simulink model "eqgraph"  (R2025b)
settings: Solver=FixedStepDiscrete  StartTime=0.0  StopTime=inf  RelTol=1e-3
undefined symbols (not defined in the file): Gain1_rt, Gain2_rt, Gain3_rt, Gain4_rt, Gain5_rt, Gain6_rt, Gain7_rt, Gain_rt
settings Model: Creator=linogarciamorales  LastModifiedBy=linogarciamorales
settings OptimizationCC: EnhancedBackFolding=on  PassReuseOutputArgsAs=Individual arguments  ZeroExternalMemoryAtStartup=off  ZeroInternalMemoryAtStartup=off  OptimizeBlockOrder=speed  DifferentSizesBufferReuse=on  OptimizationCustomize=off  EfficientTunableParamExpr=on
settings DebuggingCC: ParameterTunabilityLossMsg=error
settings HardwareCC: ProdBitPerPointer=32.0  ProdBitPerSizeT=32.0  ProdBitPerPtrDiffT=32.0  ProdLargestAtomicFloat=None  ProdIntDivRoundTo=Undefined  ProdEndianess=Unspecified  ProdWordSize=32.0  ProdHWDeviceType=Generic->32-bit Embedded Processor
settings SFSimCC: MATLABDynamicMemAlloc=off
settings RTWCC: SystemTargetFile=ert.tlc  GenCodeOnly=on  TemplateMakefile=ert_default_tmf  Description=Embedded Coder
settings CodeAppCC: ForceParamTrailComments=on  IgnoreCustomStorageClasses=off  OperatorAnnotations=on  SimulinkDataObjDesc=on  SFDataObjDesc=on  InsertBlockDesc=on
settings ERTTargetCC: InlinedParameterPlacement=Hierarchical  ERTCustomFileTemplate=example_file_process.tlc  TargetLangStandard=C99 (ISO)  SupportNonInlinedSFcns=on

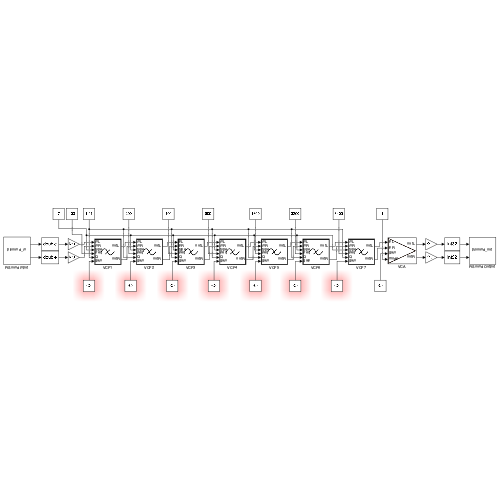
[thumbnail: Simulink's stored preview of the top-level diagram]
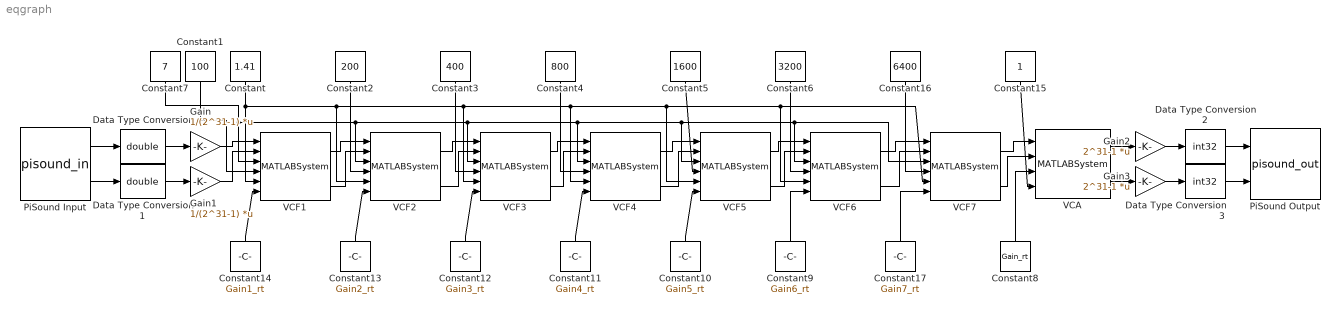
== system eqgraph ==
  Constant : Constant  Value=1.41  OutDataTypeStr=double
  Constant1 : Constant  Value=100  OutDataTypeStr=double
  Constant10 : Constant  Value=Gain5_rt  OutDataTypeStr=double
  Constant11 : Constant  Value=Gain4_rt  OutDataTypeStr=double
  Constant12 : Constant  Value=Gain3_rt  OutDataTypeStr=double
  Constant13 : Constant  Value=Gain2_rt  OutDataTypeStr=double
  Constant14 : Constant  Value=Gain1_rt  OutDataTypeStr=double
  Constant15 : Constant  OutDataTypeStr=uint8
  Constant16 : Constant  Value=6400  OutDataTypeStr=double
  Constant17 : Constant  Value=Gain7_rt  OutDataTypeStr=double
  Constant2 : Constant  Value=200  OutDataTypeStr=double
  Constant3 : Constant  Value=400  OutDataTypeStr=double
  Constant4 : Constant  Value=800  OutDataTypeStr=double
  Constant5 : Constant  Value=1600  OutDataTypeStr=double
  Constant6 : Constant  Value=3200  OutDataTypeStr=double
  Constant7 : Constant  Value=7  OutDataTypeStr=uint8
  Constant8 : Constant  Value=Gain_rt  OutDataTypeStr=double
  Constant9 : Constant  Value=Gain6_rt  OutDataTypeStr=double
  Data Type Conversion : DataTypeConversion  OutDataTypeStr=double  SaturateOnIntegerOverflow=off  RndMeth=Floor
  Data Type Conversion1 : DataTypeConversion  OutDataTypeStr=double  SaturateOnIntegerOverflow=off  RndMeth=Floor
  Data Type Conversion2 : DataTypeConversion  OutDataTypeStr=int32  SaturateOnIntegerOverflow=off  RndMeth=Floor
  Data Type Conversion3 : DataTypeConversion  OutDataTypeStr=int32  SaturateOnIntegerOverflow=off  RndMeth=Floor
  Gain : Gain  Gain=1/(2^31-1)  Multiplication=Matrix(K*u)
  Gain1 : Gain  Gain=1/(2^31-1)  Multiplication=Matrix(K*u)
  Gain2 : Gain  Gain=2^31-1  Multiplication=Matrix(K*u)
  Gain3 : Gain  Gain=2^31-1  Multiplication=Matrix(K*u)
  PiSound Input : S-Function  FunctionName=pisound_in  Parameters=48000, 128, 0  SFunctionDeploymentMode=off  EnableBusSupport=off
  PiSound Output : S-Function  FunctionName=pisound_out  Parameters=48000, 128, 0  SFunctionDeploymentMode=off  EnableBusSupport=off
  VCA : MATLABSystem  System=vca_sys  N=128  Fs=48000  bypass=uint8(0)  SimulateUsing=Code generation
      mask Type: vca_sys
  VCF1 : MATLABSystem  InitFcn=|  System=vcf_sys  N=128  Fs=48000  bypass=uint8(0)  SimulateUsing=Code generation
      | Type_rt = uint8(1);   % 1..7
      | Freq_rt = 1000;       % Hz
      | Q_rt    = 0.707;
      | Gain_rt = 0;          % dB
      mask Type: vcf_sys
  VCF2 : MATLABSystem  InitFcn=|  System=vcf_sys  N=128  Fs=48000  bypass=uint8(0)  SimulateUsing=Code generation
      | Type_rt = uint8(1);   % 1..7
      | Freq_rt = 1000;       % Hz
      | Q_rt    = 0.707;
      | Gain_rt = 0;          % dB
      mask Type: vcf_sys
  VCF3 : MATLABSystem  InitFcn=|  System=vcf_sys  N=128  Fs=48000  bypass=uint8(0)  SimulateUsing=Code generation
      | Type_rt = uint8(1);   % 1..7
      | Freq_rt = 1000;       % Hz
      | Q_rt    = 0.707;
      | Gain_rt = 0;          % dB
      mask Type: vcf_sys
  VCF4 : MATLABSystem  InitFcn=|  System=vcf_sys  N=128  Fs=48000  bypass=uint8(0)  SimulateUsing=Code generation
      | Type_rt = uint8(1);   % 1..7
      | Freq_rt = 1000;       % Hz
      | Q_rt    = 0.707;
      | Gain_rt = 0;          % dB
      mask Type: vcf_sys
  VCF5 : MATLABSystem  InitFcn=|  System=vcf_sys  N=128  Fs=48000  bypass=uint8(0)  SimulateUsing=Code generation
      | Type_rt = uint8(1);   % 1..7
      | Freq_rt = 1000;       % Hz
      | Q_rt    = 0.707;
      | Gain_rt = 0;          % dB
      mask Type: vcf_sys
  VCF6 : MATLABSystem  InitFcn=|  System=vcf_sys  N=128  Fs=48000  bypass=uint8(0)  SimulateUsing=Code generation
      | Type_rt = uint8(1);   % 1..7
      | Freq_rt = 1000;       % Hz
      | Q_rt    = 0.707;
      | Gain_rt = 0;          % dB
      mask Type: vcf_sys
  VCF7 : MATLABSystem  InitFcn=|  System=vcf_sys  N=128  Fs=48000  bypass=uint8(0)  SimulateUsing=Code generation
      | Type_rt = uint8(1);   % 1..7
      | Freq_rt = 1000;       % Hz
      | Q_rt    = 0.707;
      | Gain_rt = 0;          % dB
      mask Type: vcf_sys
  wires:
  PiSound Input/1 -> Data Type Conversion/1
  PiSound Input/2 -> Data Type Conversion1/1
  Data Type Conversion/1 -> Gain/1
  Data Type Conversion1/1 -> Gain1/1
  Gain2/1 -> Data Type Conversion2/1
  Gain3/1 -> Data Type Conversion3/1
  Data Type Conversion2/1 -> PiSound Output/1
  Data Type Conversion3/1 -> PiSound Output/2
  VCF1/2 -> VCF2/2
  VCF4/2 -> VCF5/2
  VCF4/1 -> VCF5/1
  VCF5/1 -> VCF6/1
  VCF3/1 -> VCF4/1
  VCF3/2 -> VCF4/2
  Gain/1 -> VCF1/1
  Gain1/1 -> VCF1/2
  VCF1/1 -> VCF2/1
  Constant/1 -> VCF1/5, VCF3/5, VCF7/5, VCF6/5, VCF5/5, VCF4/5, VCF2/5
  VCF2/1 -> VCF3/1
  VCF2/2 -> VCF3/2
  VCF5/2 -> VCF6/2
  Constant1/1 -> VCF1/4
  Constant2/1 -> VCF2/4
  Constant3/1 -> VCF3/4
  Constant4/1 -> VCF4/4
  Constant5/1 -> VCF5/4
  Constant6/1 -> VCF6/4
  Constant7/1 -> VCF1/3, VCF2/3, VCF3/3, VCF4/3, VCF6/3, VCF7/3, VCF5/3
  Constant8/1 -> VCA/3
  Constant9/1 -> VCF6/6
  Constant10/1 -> VCF5/6
  Constant11/1 -> VCF4/6
  Constant12/1 -> VCF3/6
  Constant13/1 -> VCF2/6
  Constant14/1 -> VCF1/6
  Constant15/1 -> VCA/4
  Constant17/1 -> VCF7/6
  Constant16/1 -> VCF7/4
  VCF6/2 -> VCF7/2
  VCF6/1 -> VCF7/1
  VCF7/1 -> VCA/1
  VCF7/2 -> VCA/2
  VCA/1 -> Gain2/1
  VCA/2 -> Gain3/1
